simulink model "Controlador_PID"  (R2015a)
settings: Solver=ode45  StartTime=0.0  StopTime=10  RelTol=1e-3
libraries: simulink x5
settings Model: Creator=Henry Alberto  LastModifiedBy=Henry Alberto

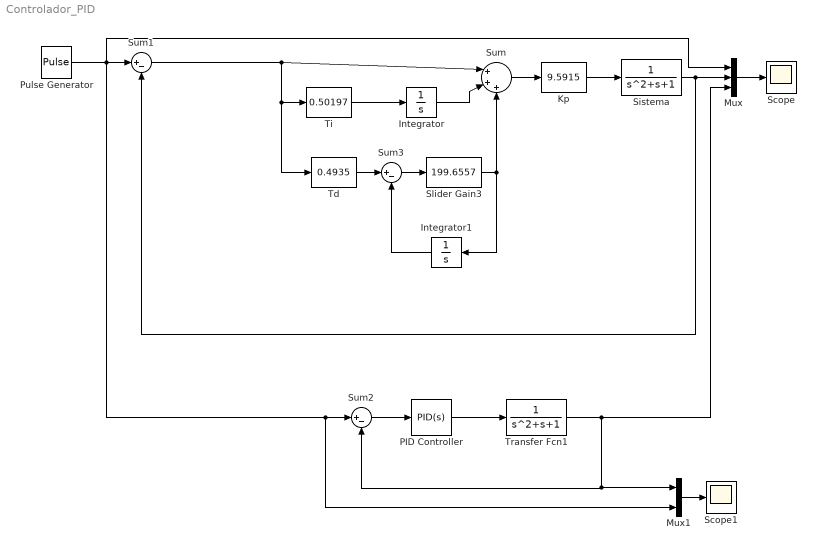
== system Controlador_PID ==
  Integrator : Integrator
  Integrator1 : Integrator
  Kp : simulink/Math Operations/Slider Gain  low=0  gain=9.5915  high=1000
  Mux : Mux  Inputs=3
  Mux1 : Mux  Inputs=2
  PID Controller : simulink/Continuous/PID Controller  Controller=PID  TimeDomain=Continuous-time  SampleTime=-1  IntegratorMethod=Forward Euler  FilterMethod=Forward Euler  Form=Ideal  UseFilter=on  ControllerParametersSource=internal  P=2.44388162448714  I=0.559065176144384  D=0.440845353041874  N=199.655710994834  InitialConditionSource=internal  InitialConditionForIntegrator=0  InitialConditionForFilter=0  ExternalReset=none  LimitOutput=off  UpperSaturationLimit=inf  LowerSaturationLimit=-inf  LinearizeAsGain=on  AntiWindupMode=none  Kb=1  TrackingMode=off  Kt=1  PParamMin=[]  PParamMax=[]  IParamMin=[]  IParamMax=[]  DParamMin=[]  DParamMax=[]  NParamMin=[]  NParamMax=[]  KbParamMin=[]  KbParamMax=[]  KtParamMin=[]  KtParamMax=[]  POutMin=[]  POutMax=[]  IOutMin=[]  IOutMax=[]  DOutMin=[]  DOutMax=[]  NOutMin=[]  NOutMax=[]  KbOutMin=[]  KbOutMax=[]  KtOutMin=[]  KtOutMax=[]  IntegratorOutMin=[]  IntegratorOutMax=[]  FilterOutMin=[]  FilterOutMax=[]  SumOutMin=[]  SumOutMax=[]  SumI1OutMin=[]  SumI1OutMax=[]  SumI2OutMin=[]  SumI2OutMax=[]  SumI3OutMin=[]  SumI3OutMax=[]  SumDOutMin=[]  SumDOutMax=[]  SaturationOutMin=[]  SaturationOutMax=[]  IntegratorContinuousStateAttributes=''  IntegratorStateMustResolveToSignalObject=off  IntegratorRTWStateStorageClass=Auto  FilterContinuousStateAttributes=''  FilterStateMustResolveToSignalObject=off  FilterRTWStateStorageClass=Auto  DifferentiatorICPrevScaledInput=0  DifferentiatorOutMin=[]  DifferentiatorOutMax=[]
  Pulse Generator : DiscretePulseGenerator  PulseType=Time based  Period=10  PulseWidth=50
  Scope : Scope
      settings: YMin=-0.25  YMax=1.25
  Scope1 : Scope
  "Sistema " : TransferFcn  Denominator=[1 1 1]
  Slider Gain3 : simulink/Math Operations/Slider Gain  low=0  gain=199.6557  high=500
  Sum : Sum  Inputs=|+++
  Sum1 : Sum  Inputs=|+-
  Sum2 : Sum  Inputs=|+-
  Sum3 : Sum  Inputs=|+-
  Td : simulink/Math Operations/Slider Gain  low=0  gain=0.4935  high=2
  Ti : simulink/Math Operations/Slider Gain  low=0  gain=0.50197  high=20
  Transfer Fcn1 : TransferFcn  Denominator=[1 1 1]
  wires:
  Integrator/1 -> Sum/2
  Ti/1 -> Integrator/1
  Sum1/1 -> Td/1, Ti/1, Sum/1
  "Sistema "/1 -> Mux/2, Sum1/2
  Mux/1 -> Scope/1
  PID Controller/1 -> Transfer Fcn1/1
  Pulse Generator/1 -> Mux/1, Mux1/2, Sum2/1, Sum1/1
  Sum2/1 -> PID Controller/1
  Transfer Fcn1/1 -> Mux1/1, Sum2/2, Mux/3
  Mux1/1 -> Scope1/1
  Kp/1 -> "Sistema "/1
  Sum/1 -> Kp/1
  Td/1 -> Sum3/1
  Sum3/1 -> Slider Gain3/1
  Slider Gain3/1 -> Integrator1/1, Sum/3
  Integrator1/1 -> Sum3/2
